simulink model "Display_Demo"  (R2022a)
settings: Solver=ode5  StartTime=0.0  StopTime=10.0  FixedStep=.01  RelTol=1e-3
values from neighbouring files (symbols this model uses):
  DREF_airspeed_kts_pilot = uint8('sim/cockpit2/gauges/indicators/airspeed_kts_pilot')    [DREF_init.m]    (also in xplane_UDP_Demo.m)
  DREF_ID_str = [uint8('DREF') 0x00]    [DREF_init.m]    (also in xplane_UDP_Demo.m)
  VEHX_ID_str = [uint8('VEHX') 0x00]    [DREF_init.m]    (also in xplane_UDP_Demo.m)
undefined symbols (not defined in the file or in its folder): Standard_Devices, UDP_Protocol
libraries: sldrtlib x3
settings Model: Creator=Jeremy  LastModifiedBy=Zi Wang
settings DebuggingCC: UnconnectedInputMsg=warning  UnconnectedOutputMsg=warning  UnconnectedLineMsg=warning
settings HardwareCC: ProdBitPerLong=64  ProdHWDeviceType=Intel->x86-64 (Linux 64)
settings RTWCC: Description=Simulink Desktop Real-Time  SystemTargetFile=sldrt.tlc  TemplateMakefile=sldrt.tmf  RTWCompilerOptimization=on  DLArmComputeVersion=19.05
settings CodeAppCC: MaxIdLength=95
settings SimulinkDesktopRealTimeCC: TargetLibSuffix=_sldrt.a  TargetPreCompLibLocation=C:\Program Files\MATLAB\R2022a\toolbox\sldrt\lib\win64

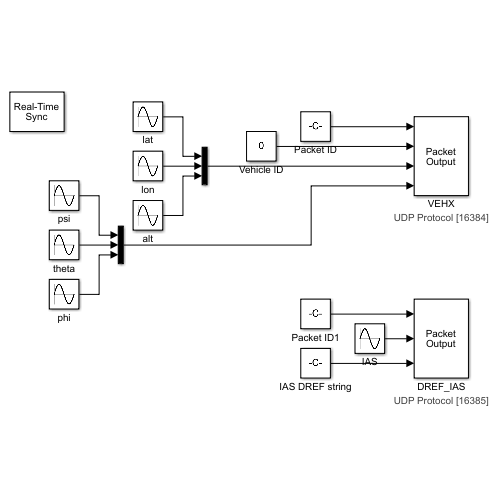
[thumbnail: Simulink's stored preview of the top-level diagram]
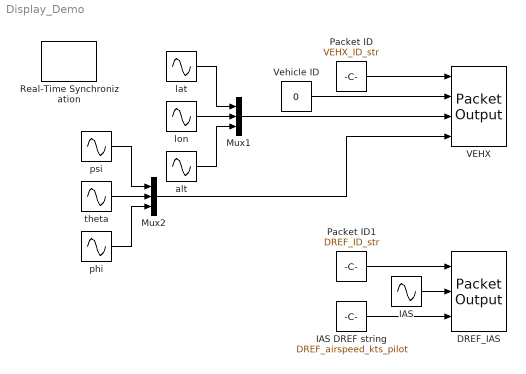
== system Display_Demo ==
  DREF_IAS : sldrtlib/Packet Output  SampleTime=0.01  MaxMissedTicks=10  ShowMissedTicks=off  YieldWhenWaiting=off  DrvName=Standard_Devices/UDP_Protocol  DrvAddress=16385  DrvOptions=[0 49000 49 50 55 46 48 46 48 46 49 0 0 0 0 0 0 0 0 0 0 0 0 0 0 0 0 0 0 0 0 0 0 0 0 0 0 0 0 0 0 0 0 0 0 0 0 0 0 0 0 0 0 0 0 0 0 0 0 0 0 0 0 0 0 0 0 0 0 0 0 0 0 0 0 0 0 0 0 0 0 0 0 0 0 0 0 0 0 0 0 0 0 0 0 0 0 0 0 0 0 0 0 0 0 0 0 0 0 0 0 0 0 0 0 0 0 0 0 0 0 0 0 0 0 0 0 0 0 0 0 0 0 0 0 0 0 0 0 0 0 0 0 0 0 0 0 0 0 0 0 0 0 0 0 0 0 0 0 0 0 0 0 0 0 0 0 0 0 0 0 0 0 0 0 0 0 0 0 0 0 0 0 0 0 0 0 0 0 0 0 0 0 0 0 0 0 0 0 0 0 0 0 0 0 0 0 0 0 0 0 0 0 0 0 0 0 0 0 0 0 0 0 0 0 0 0 0 0 0 0 0 0 0 0 0 0 0 0 0 0 0 0 0 0 0 0 0 0 0 0 0 0 0 0 0]  PacketSize=509  DataTypes={'5*uint8', '1*single','500*uint8'}  ShowReady=off  ShowError=off  PacketID=1  ByteOrder=1  InitialValue=[]  FinalValue=[]
      settings: AttributesFormatString=UDP Protocol [16385]
  IAS : Sin  Amplitude=50  Bias=100  Frequency=.5  Phase=pi/2  SampleTime=0
  IAS DREF string : Constant  Value=DREF_airspeed_kts_pilot
  Mux1 : Mux  Inputs=3
  Mux2 : Mux  Inputs=3
  Packet ID : Constant  Value=VEHX_ID_str
  Packet ID1 : Constant  Value=DREF_ID_str
  Real-Time Synchronization : sldrtlib/Real-Time Synchronization  SampleTime=0.1  MaxMissedTicks=10  ShowMissedTicks=off  YieldWhenWaiting=off
  VEHX : sldrtlib/Packet Output  SampleTime=0.01  MaxMissedTicks=10  ShowMissedTicks=off  YieldWhenWaiting=off  DrvName=Standard_Devices/UDP_Protocol  DrvAddress=16384  DrvOptions=[0 49000 49 50 55 46 48 46 48 46 49 0 0 0 0 0 0 0 0 0 0 0 0 0 0 0 0 0 0 0 0 0 0 0 0 0 0 0 0 0 0 0 0 0 0 0 0 0 0 0 0 0 0 0 0 0 0 0 0 0 0 0 0 0 0 0 0 0 0 0 0 0 0 0 0 0 0 0 0 0 0 0 0 0 0 0 0 0 0 0 0 0 0 0 0 0 0 0 0 0 0 0 0 0 0 0 0 0 0 0 0 0 0 0 0 0 0 0 0 0 0 0 0 0 0 0 0 0 0 0 0 0 0 0 0 0 0 0 0 0 0 0 0 0 0 0 0 0 0 0 0 0 0 0 0 0 0 0 0 0 0 0 0 0 0 0 0 0 0 0 0 0 0 0 0 0 0 0 0 0 0 0 0 0 0 0 0 0 0 0 0 0 0 0 0 0 0 0 0 0 0 0 0 0 0 0 0 0 0 0 0 0 0 0 0 0 0 0 0 0 0 0 0 0 0 0 0 0 0 0 0 0 0 0 0 0 0 0 0 0 0 0 0 0 0 0 0 0 0 0 0 0 0 0 0 0]  PacketSize=45  DataTypes={'5*uint8', '1*int32','3*double','3*single'}  ShowReady=off  ShowError=off  PacketID=1  ByteOrder=1  InitialValue=[]  FinalValue=[]
      settings: AttributesFormatString=UDP Protocol [16384]
  Vehicle ID : Constant  Value=0
  alt : Sin  Amplitude=1000  Bias=2000  Frequency=.5  SampleTime=0
  lat : Sin  Amplitude=.05  Bias=-33  Frequency=.5  Phase=pi/2  SampleTime=0
  lon : Sin  Amplitude=.05  Bias=151  Frequency=.5  SampleTime=0
  phi : Sin  Amplitude=90  Frequency=.5  SampleTime=0
  psi : Sin  Amplitude=90  Frequency=.5  SampleTime=0
  theta : Sin  Amplitude=90  Frequency=.5  SampleTime=0
  wires:
  Mux1/1 -> VEHX/3
  Packet ID/1 -> VEHX/1
  Vehicle ID/1 -> VEHX/2
  theta/1 -> Mux2/2
  phi/1 -> Mux2/3
  lat/1 -> Mux1/1
  lon/1 -> Mux1/2
  alt/1 -> Mux1/3
  Mux2/1 -> VEHX/4
  psi/1 -> Mux2/1
  Packet ID1/1 -> DREF_IAS/1
  IAS DREF string/1 -> DREF_IAS/3
  IAS/1 -> DREF_IAS/2
